simulink model "Baxter_PID"  (R2015b)
settings: Solver=FixedStepDiscrete  StartTime=0.0  StopTime=40  FixedStep=0.04  RelTol=1e-3
InitFcn:
  | initGoals
StopFcn:
  | stopBaxter
model workspace (MAT data in the model file):
  SL_ROS_VariableLengthArrays_MaxSizes.CommonInfo.ArrayTruncateAction = 'EmitWarning'
  SL_ROS_VariableLengthArrays_MaxSizes.MsgTypeMap = containers.Map
  SL_ROS_VariableLengthArrays_MaxSizes.MsgTypeMap.serialization.keys = {'baxter_core_msgs/JointCommand', 'sensor_msgs/JointState'}
  SL_ROS_VariableLengthArrays_MaxSizes.MsgTypeMap.serialization.values{1}(1).PropertyName = 'Command'
  SL_ROS_VariableLengthArrays_MaxSizes.MsgTypeMap.serialization.values{1}(1).DataType = 'double'
  SL_ROS_VariableLengthArrays_MaxSizes.MsgTypeMap.serialization.values{1}(1).MaxLength = 7
  SL_ROS_VariableLengthArrays_MaxSizes.MsgTypeMap.serialization.values{1}(2).PropertyName = 'Names'
  SL_ROS_VariableLengthArrays_MaxSizes.MsgTypeMap.serialization.values{1}(2).DataType = 'std_msgs/String'
  SL_ROS_VariableLengthArrays_MaxSizes.MsgTypeMap.serialization.values{1}(2).MaxLength = 7
  SL_ROS_VariableLengthArrays_MaxSizes.MsgTypeMap.serialization.values{2}(1).PropertyName = 'Name'
  SL_ROS_VariableLengthArrays_MaxSizes.MsgTypeMap.serialization.values{2}(1).DataType = 'std_msgs/String'
  SL_ROS_VariableLengthArrays_MaxSizes.MsgTypeMap.serialization.values{2}(1).MaxLength = 128
  SL_ROS_VariableLengthArrays_MaxSizes.MsgTypeMap.serialization.values{2}(2).PropertyName = 'Position'
  SL_ROS_VariableLengthArrays_MaxSizes.MsgTypeMap.serialization.values{2}(2).DataType = 'double'
  SL_ROS_VariableLengthArrays_MaxSizes.MsgTypeMap.serialization.values{2}(2).MaxLength = 128
  SL_ROS_VariableLengthArrays_MaxSizes.MsgTypeMap.serialization.values{2}(3).PropertyName = 'Velocity'
  SL_ROS_VariableLengthArrays_MaxSizes.MsgTypeMap.serialization.values{2}(3).DataType = 'double'
  SL_ROS_VariableLengthArrays_MaxSizes.MsgTypeMap.serialization.values{2}(3).MaxLength = 128
  SL_ROS_VariableLengthArrays_MaxSizes.MsgTypeMap.serialization.values{2}(4).PropertyName = 'Effort'
  SL_ROS_VariableLengthArrays_MaxSizes.MsgTypeMap.serialization.values{2}(4).DataType = 'double'
  SL_ROS_VariableLengthArrays_MaxSizes.MsgTypeMap.serialization.values{2}(4).MaxLength = 128
  SL_ROS_VariableLengthArrays_MaxSizes.MsgTypeMap.serialization.uniformity = 0
  SL_ROS_VariableLengthArrays_MaxSizes.MsgTypeMap.serialization.keyType = 'char'
  SL_ROS_VariableLengthArrays_MaxSizes.MsgTypeMap.serialization.valueType = 'any'
undefined symbols (not defined in the file or in its folder): robotics
libraries: simulink x7, robotlib x6, lab3lib x1
settings Model: Creator=baxter  LastModifiedBy=Stefan
settings DataIOCC: SaveFormat=Array
settings DebuggingCC: AllowSymbolicDim=on
settings HardwareCC: ProdBitPerPointer=32  ProdLargestAtomicFloat=None  ProdIntDivRoundTo=Undefined  ProdEndianess=Unspecified  ProdWordSize=32  ProdHWDeviceType=32-bit Generic
settings GRTTargetCC: GeneratePreprocessorConditionals=Disable all
settings ConfigComp: CovModelRefEnable=Off

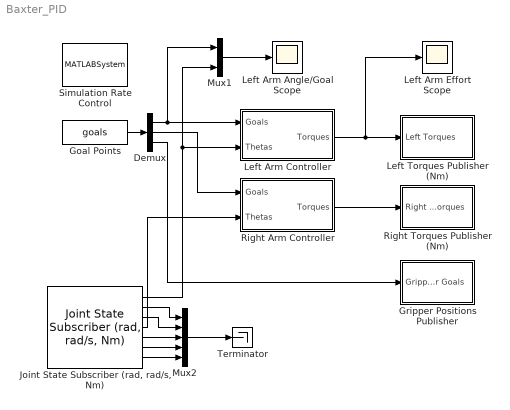
== system Baxter_PID ==
  Demux : Demux  Outputs=3
  Goal Points : FromWorkspace  VariableName=goals  SampleTime=0  Interpolate=off  OutputAfterFinalValue=Holding final value
  Gripper Positions Publisher : Subsystem  mask(Left Joint Torques){}
      mask help: Outputs the joint position commands to the left and right grippers of either the simulated or physical Baxter robot.
  "Joint State Subscriber (rad, rad/s, Nm)" : lab3lib/Joint State Subscriber (rad, rad//s, Nm)
  Left Arm Angle/Goal Scope : Scope
  Left Arm Controller : Subsystem
  Left Arm Effort Scope : Scope
  Left Torques Publisher (Nm) : Subsystem  mask(Left Joint Torques){}
      mask help: Outputs the joint torque commands to the left arm of either the simulated or physical Baxter robot.
  Mux1 : Mux  Inputs=2
  Mux2 : Mux  Inputs=5
  Right Arm Controller : Subsystem
  Right Torques Publisher (Nm) : Subsystem  mask(Left Joint Torques){}
      mask help: Outputs the joint torque commands to the left arm of either the simulated or physical Baxter robot.
  Simulation Rate Control : MATLABSystem  System=ExampleHelperSimulationRateControl  SampleTime=0.04
      mask Type: ExampleHelperSimulationRateControl
      mask Display: disp('Rate Control');
  Terminator : Terminator
  wires:
  Left Arm Controller/1(Torques) -> Left Torques Publisher (Nm)/1(Left Torques), Left Arm Effort Scope/1
  Demux/1 -> Mux1/1, Left Arm Controller/1(Goals)
  Mux1/1 -> Left Arm Angle/Goal Scope/1
  "Joint State Subscriber (rad, rad/s, Nm)"/1 -> Left Arm Controller/2(Thetas), Mux1/2
  "Joint State Subscriber (rad, rad/s, Nm)"/2 -> Mux2/1
  "Joint State Subscriber (rad, rad/s, Nm)"/4 -> Right Arm Controller/2(Thetas)
  "Joint State Subscriber (rad, rad/s, Nm)"/5 -> Mux2/3
  "Joint State Subscriber (rad, rad/s, Nm)"/6 -> Mux2/4
  "Joint State Subscriber (rad, rad/s, Nm)"/7 -> Mux2/5
  Mux2/1 -> Terminator/1
  Goal Points/1 -> Demux/1
  Demux/2 -> Right Arm Controller/1(Goals)
  Right Arm Controller/1(Torques) -> Right Torques Publisher (Nm)/1(Right Torques)
  Demux/3 -> Gripper Positions Publisher/1(Gripper Goals)
  "Joint State Subscriber (rad, rad/s, Nm)"/3 -> Mux2/2

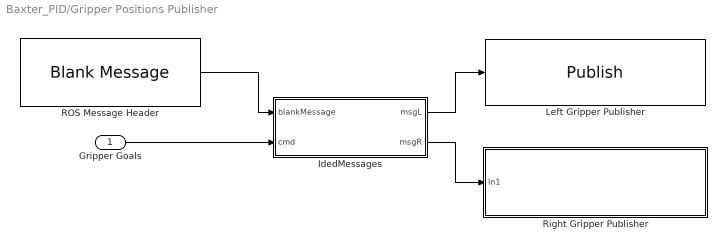
== system Baxter_PID/Gripper Positions Publisher ==
  Gripper Goals : Inport  PortDimensions=2
  IdedMessages : MATLAB Function  TreatAsAtomicUnit=on
  Left Gripper Publisher : robotlib/Publish  SourceLibraryInfo=This block requires Robotics System Toolbox  topicSource=Select from ROS network  topic=/robot/end_effector/left_gripper/command  messageType=baxter_core_msgs/EndEffectorCommand  messageQueueLength=1
  ROS Message Header : robotlib/Blank Message  SourceLibraryInfo=This block requires Robotics System Toolbox  messageType=baxter_core_msgs/EndEffectorCommand  SampleTime=inf
  Right Gripper Publisher : Subsystem  AncestorBlock=robotlib/Publish  TreatAsAtomicUnit=on  mask(ROS Publish){topicSource=Select from ROS network, topic=/robot/end_effector/right_gripper/command, messageType=baxter_core_msgs/EndEffectorCommand, outputStreamWsVar=, messageQueueLength=1}
      mask prompts: topicSource "robotics:robotslros:blockmask:TopicSourcePrompt"; topic "robotics:robotslros:blockmask:TopicPrompt"; messageType "robotics:robotslros:blockmask:MessageTypePrompt"; outputStreamWsVar "robotics:robotslros:blockmask:PublisherOutputStreamPrompt"; messageQueueLength "robotics:robotslros:blockmask:PublisherMsgQueuePrompt"
      mask help: robotics:robotslros:blockmask:PublisherDescription
      mask init:
      | robotics.slros.internal.block.PublishBlockMask.dispatch('maskInitialize', gcb);
      settings: ModelCloseFcn=robotics.slros.internal.block.PublishBlockMask.dispatch('modelCloseFcn', gcb);
      mask Help: eval('robotics.slros.internal.helpview(''rosPublishBlock'')');
      mask TypeOptions topicSource: Select from ROS network | Specify your own
      mask Callback topicSource: robotics.slros.internal.block.PublishBlockMask.dispatch('topicSourceSelect', gcb);
      mask Callback topic: robotics.slros.internal.block.PublishBlockMask.dispatch('topicEdit', gcb);
      mask TypeOptions outputStreamWsVar: SinkBlock/OutputStreamWsVar
      mask TypeOptions messageQueueLength: SinkBlock/MessageQueueLen
      mask DialogControl id_netAddrLink Prompt: robotics:robotslros:blockmask:ConfigNetworkAddrLinkText
      mask DialogControl id_netAddrLink Callback: robotics.slros.internal.block.PublishBlockMask.dispatch('configureNetworkAddrDlg', gcb);
      mask DialogControl id_topicSelectBtn Prompt: robotics:robotslros:blockmask:SelectPrompt
      mask DialogControl id_topicSelectBtn Callback: robotics.slros.internal.block.PublishBlockMask.dispatch('topicSelect', gcb);
      mask DialogControl id_msgTypeSelectBtn Prompt: robotics:robotslros:blockmask:SelectPrompt
      mask DialogControl id_msgTypeSelectBtn Callback: robotics.slros.internal.block.PublishBlockMask.dispatch('messageTypeSelect', gcb);
      mask Display:
      | color('blue');
      | text(0.2, 0.90, 'ROS', 'horizontalAlignment', 'right');
      | color('black');
      | text(0.5, 0.60, 'Publish', 'horizontalAlignment', 'center');
      | if length(topic) > 20
      |   text(0.95, 0.15, topic, 'horizontalAlignment', 'right');
      | else
      |   text(0.5, 0.15, topic, 'horizontalAlignment', 'center');
      | end
      | port_label('input', 1, 'Msg');
  wires:
  Gripper Goals/1 -> IdedMessages/2(cmd)
  ROS Message Header/1 -> IdedMessages/1(blankMessage)
  IdedMessages/1(msgL) -> Left Gripper Publisher/1
  IdedMessages/2(msgR) -> Right Gripper Publisher/1(In1)

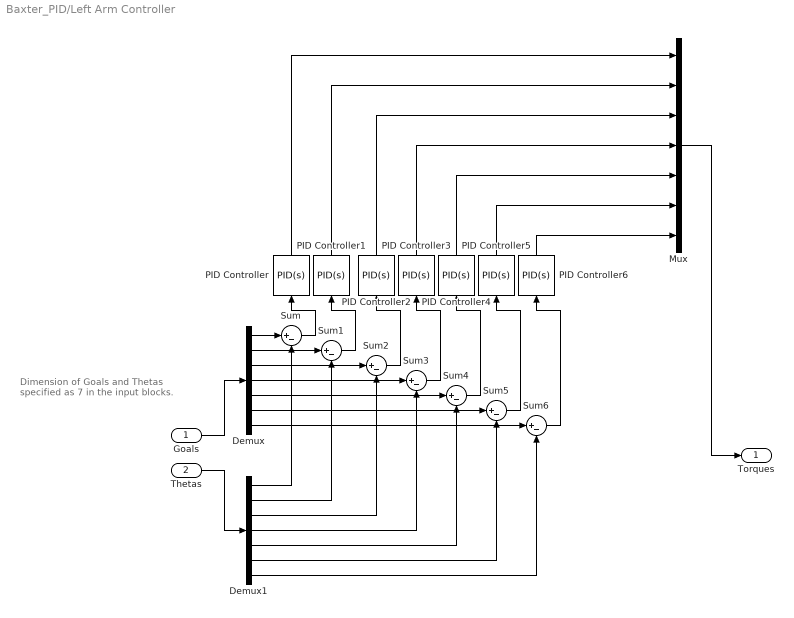
== system Baxter_PID/Left Arm Controller ==
  note: Dimension of Goals and Thetas
      | specified as 7 in the input blocks.
  Goals : Inport  PortDimensions=7
  Thetas : Inport  Port=2  PortDimensions=7
  Demux : Demux  Outputs=7
  Demux1 : Demux  Outputs=7
  Mux : Mux  Inputs=7
  PID Controller{,1..6} (7 alike) : simulink/Continuous/PID Controller  Controller=PID  TimeDomain=Continuous-time  SampleTime=-1  IntegratorMethod=Forward Euler  FilterMethod=Forward Euler  Form=Parallel  UseFilter=on  ControllerParametersSource=internal  P=1  I=1  D=0  N=100  InitialConditionSource=internal  InitialConditionForIntegrator=0  InitialConditionForFilter=0  ExternalReset=none  LimitOutput=off  UpperSaturationLimit=inf  LowerSaturationLimit=-inf  LinearizeAsGain=on  AntiWindupMode=none  Kb=1  TrackingMode=off  Kt=1  PParamMin=[]  PParamMax=[]  IParamMin=[]  IParamMax=[]  DParamMin=[]  DParamMax=[]  NParamMin=[]  NParamMax=[]  KbParamMin=[]  KbParamMax=[]  KtParamMin=[]  KtParamMax=[]  POutMin=[]  POutMax=[]  IOutMin=[]  IOutMax=[]  DOutMin=[]  DOutMax=[]  NOutMin=[]  NOutMax=[]  KbOutMin=[]  KbOutMax=[]  KtOutMin=[]  KtOutMax=[]  IntegratorOutMin=[]  IntegratorOutMax=[]  FilterOutMin=[]  FilterOutMax=[]  SumOutMin=[]  SumOutMax=[]  SumI1OutMin=[]  SumI1OutMax=[]  SumI2OutMin=[]  SumI2OutMax=[]  SumI3OutMin=[]  SumI3OutMax=[]  SumDOutMin=[]  SumDOutMax=[]  SaturationOutMin=[]  SaturationOutMax=[]  IntegratorContinuousStateAttributes=''  IntegratorStateMustResolveToSignalObject=off  IntegratorRTWStateStorageClass=Auto  FilterContinuousStateAttributes=''  FilterStateMustResolveToSignalObject=off  FilterRTWStateStorageClass=Auto  DifferentiatorICPrevScaledInput=0  DifferentiatorOutMin=[]  DifferentiatorOutMax=[]
  Sum{,1..6} (7 alike) : Sum  Inputs=|+-
  Torques : Outport
  wires:
  Thetas/1 -> Demux1/1
  Goals/1 -> Demux/1
  Demux/1 -> Sum/1
  Demux/2 -> Sum1/1
  Demux/3 -> Sum2/1
  Demux/4 -> Sum3/1
  Demux/5 -> Sum4/1
  Demux/6 -> Sum5/1
  Demux/7 -> Sum6/1
  Demux1/1 -> Sum/2
  Demux1/2 -> Sum1/2
  Demux1/3 -> Sum2/2
  Demux1/4 -> Sum3/2
  Demux1/5 -> Sum4/2
  Demux1/6 -> Sum5/2
  Demux1/7 -> Sum6/2
  Sum/1 -> PID Controller/1
  PID Controller/1 -> Mux/1
  Mux/1 -> Torques/1
  Sum1/1 -> PID Controller1/1
  Sum2/1 -> PID Controller2/1
  Sum3/1 -> PID Controller3/1
  Sum4/1 -> PID Controller4/1
  Sum5/1 -> PID Controller5/1
  Sum6/1 -> PID Controller6/1
  PID Controller1/1 -> Mux/2
  PID Controller2/1 -> Mux/3
  PID Controller3/1 -> Mux/4
  PID Controller4/1 -> Mux/5
  PID Controller5/1 -> Mux/6
  PID Controller6/1 -> Mux/7

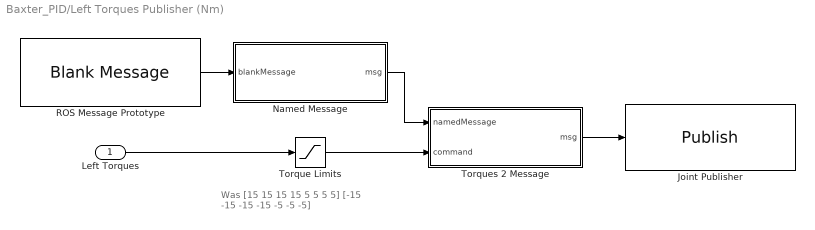
== system Baxter_PID/Left Torques Publisher (Nm) ==
  note: Was [15 15 15 15 5 5 5 5]
      | [-15 -15 -15 -15 -5 -5 -5]
  Left Torques : Inport  PortDimensions=7
  Joint Publisher : robotlib/Publish  SourceLibraryInfo=This block requires Robotics System Toolbox  topicSource=Select from ROS network  topic=/robot/limb/left/joint_command  messageType=baxter_core_msgs/JointCommand  messageQueueLength=1
  Named Message : MATLAB Function  TreatAsAtomicUnit=on
  ROS Message Prototype : robotlib/Blank Message  SourceLibraryInfo=This block requires Robotics System Toolbox  messageType=baxter_core_msgs/JointCommand  SampleTime=inf
  Torque Limits : Saturate  UpperLimit=[5 5 5 5 5 5 5]  LowerLimit=[-5 -5 -5 -5 -5 -5 -5]
  Torques 2 Message : MATLAB Function  AncestorBlock=lab3lib/Torques 2 Message  TreatAsAtomicUnit=on
  wires:
  Torques 2 Message/1(msg) -> Joint Publisher/1
  Named Message/1(msg) -> Torques 2 Message/1(namedMessage)
  ROS Message Prototype/1 -> Named Message/1(blankMessage)
  Left Torques/1 -> Torque Limits/1
  Torque Limits/1 -> Torques 2 Message/2(command)

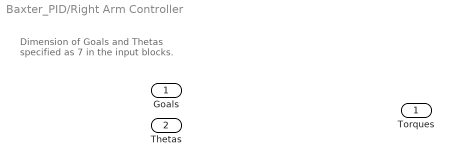
== system Baxter_PID/Right Arm Controller ==
  note: Dimension of Goals and Thetas
      | specified as 7 in the input blocks.
  Goals : Inport  PortDimensions=7
  Thetas : Inport  Port=2  PortDimensions=7
  Torques : Outport

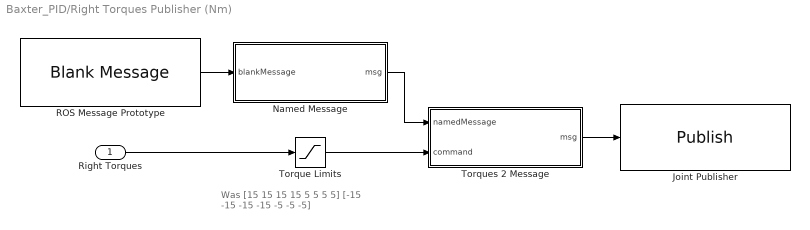
== system Baxter_PID/Right Torques Publisher (Nm) ==
  note: Was [15 15 15 15 5 5 5 5]
      | [-15 -15 -15 -15 -5 -5 -5]
  Right Torques : Inport  PortDimensions=7
  Joint Publisher : robotlib/Publish  SourceLibraryInfo=This block requires Robotics System Toolbox  topicSource=Select from ROS network  topic=/robot/limb/right/joint_command  messageType=baxter_core_msgs/JointCommand  messageQueueLength=1
  Named Message : MATLAB Function  TreatAsAtomicUnit=on
  ROS Message Prototype : robotlib/Blank Message  SourceLibraryInfo=This block requires Robotics System Toolbox  messageType=baxter_core_msgs/JointCommand  SampleTime=inf
  Torque Limits : Saturate  UpperLimit=[5 5 5 5 5 5 5]  LowerLimit=[-5 -5 -5 -5 -5 -5 -5]
  Torques 2 Message : MATLAB Function  AncestorBlock=lab3lib/Torques 2 Message  TreatAsAtomicUnit=on
  wires:
  Right Torques/1 -> Torque Limits/1
  ROS Message Prototype/1 -> Named Message/1(blankMessage)
  Named Message/1(msg) -> Torques 2 Message/1(namedMessage)
  Torques 2 Message/1(msg) -> Joint Publisher/1
  Torque Limits/1 -> Torques 2 Message/2(command)

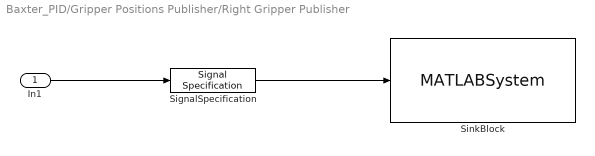
== system Baxter_PID/Gripper Positions Publisher/Right Gripper Publisher ==
  In1 : Inport  LockScale=on
  SignalSpecification : SignalSpecification  OutDataTypeStr=Bus: SL_Bus_Baxter_PID_baxter_core_msgs_EndEffectorCommand  BusOutputAsStruct=on
      settings: LockScale=on
  SinkBlock : MATLABSystem  InitFcn=robotics.slros.internal.block.PublishBlockMask.dispatch('sysobjInitFcn', gcb);  System=robotics.slros.internal.block.Publisher  ROSTopic=/robot/end_effector/right_gripper/command  ROSMessageType=baxter_core_msgs/EndEffectorCommand  MessageQueueLen=messageQueueLength  SLBusName=SL_Bus_Baxter_PID_baxter_core_msgs_EndEffectorCommand  ModelName=Baxter_PID  BlockId=Pub_Baxter_PID_609  SimulateUsing=Interpreted execution
      mask Type: robotics.slros.internal.block.Publisher
      mask Display:
      | disp('Publisher');
      | port_label('input',1,'busstruct');
  wires:
  In1/1 -> SignalSpecification/1
  SignalSpecification/1 -> SinkBlock/1

== matlab function Baxter_PID/Left Torques Publisher (Nm)/Named Message ==
  data: blankMessage input; msg output SL_Bus_Baxter_PID_baxter_core_msgs_JointCommand
function msg = namedMsg(blankMessage)
%#codegen

%% Create a blank Baxter JointCommand message, fill with data
msg=blankMessage; % Get message prototype from simulink BlankMessage block

%% Handle Names field
% What each joint in the command message is - just controlling the left arm
% Shoulder 0,1, elbow 0,1, wrist 0,1,2 - moving away from shoulder joint
names={'left_s0','left_s1','left_e0','left_e1','left_w0','left_w1','left_w2'};
msg = writeNames(names,msg);

% Set Mode to torque control
msg.Mode=int32(3); % position mode 1, velocity mode 2, torque mode 3

end

== matlab function Baxter_PID/Gripper Positions Publisher/IdedMessages ==
  data: blankMessage input; msgL output Bus: SL_Bus_Baxter_PID_baxter_core_msgs_EndEffectorCommand; cmd input; msgR output Bus: SL_Bus_Baxter_PID_baxter_core_msgs_EndEffectorCommand
function [msgL,msgR] = namedMsg(blankMessage, cmd)
%#codegen

%% Copy a blank Baxter JointCommand message, fill with data
msg = blankMessage; % Get message prototype from simulink BlankMessage block
msg.Id = uint32(65538);
msg.Args(1:2) = uint8('{}');
msg.Args_SL_Info.CurrentLength = uint32(2);
msg.Sequence = uint32(1);
msg.Sender(1:4) = uint8('host');
msg.Sender_SL_Info.CurrentLength = uint32(4);
msgL = msg; % Copy what's the same
msgR = msg; % Copy what's the same

%% Handle Names field
% What each joint in the command message is - just controlling the grippers
% names={'l_gripper_l_finger_joint'}; %,'r_gripper_l_finger_joint'};
% msg = writeNames(names,msg);
if cmd(1) < 0.015
    msgL.Command(1:4) = uint8('grip');
    msgL.Command_SL_Info.CurrentLength = uint32(4);
else
    msgL.Command(1:7) = uint8('release');
    msgL.Command_SL_Info.CurrentLength = uint32(7);
end

if cmd(2) < 0.015
    msgR.Command(1:4) = uint8('grip');
    msgR.Command_SL_Info.CurrentLength = uint32(4);
else
    msgR.Command(1:7) = uint8('release');
    msgR.Command_SL_Info.CurrentLength = uint32(7);
end

end

== matlab function Baxter_PID/Right Torques Publisher (Nm)/Named Message ==
  data: blankMessage input; msg output Bus: SL_Bus_Baxter_PID_baxter_core_msgs_JointCommand
function msg = namedMsg(blankMessage)
%#codegen

%% Create a blank Baxter JointCommand message, fill with data
msg=blankMessage; % Get message prototype from simulink BlankMessage block

%% Handle Names field
% What each joint in the command message is - just controlling the right arm
% Shoulder 0,1, elbow 0,1, wrist 0,1,2 - moving away from shoulder joint
names={'right_s0','right_s1','right_e0','right_e1','right_w0','right_w1','right_w2'};
msg = writeNames(names,msg);

% Set Mode to torque control
msg.Mode=int32(3); % position mode 1, velocity mode 2, torque mode 3

end

== matlab function Baxter_PID/Left Torques Publisher (Nm)/Torques 2 Message ==
  data: namedMessage input; command input; msg output Bus: SL_Bus_Baxter_PID_baxter_core_msgs_JointCommand
function msg = cmdMsg(namedMessage, command)
%#codegen

%% Create a blank Baxter JointCommand message, fill with data
msg=namedMessage; % Get message prototype from simulink BlankMessage block

%% Handle Command field
msg.Command(1:length(command))=command; %the position you want it to be
msg.Command_SL_Info.CurrentLength=uint32(length(command)); %length of torques

end

== matlab function Baxter_PID/Right Torques Publisher (Nm)/Torques 2 Message ==
  data: namedMessage input; command input; msg output Bus: SL_Bus_Baxter_PID_baxter_core_msgs_JointCommand
function msg = cmdMsg(namedMessage, command)
%#codegen

%% Create a blank Baxter JointCommand message, fill with data
msg=namedMessage; % Get message prototype from simulink BlankMessage block

%% Handle Command field
msg.Command(1:length(command))=command; %the position you want it to be
msg.Command_SL_Info.CurrentLength=uint32(length(command)); %length of torques

end
